simulink model "Experiment_4"  (R2018b)
settings: Solver=VariableStepAuto  StartTime=0.0  StopTime=2  RelTol=1e-3
libraries: dsparch4 x1, commsynccomp2 x1
settings Model: Creator=sangh  LastModifiedBy=sangh

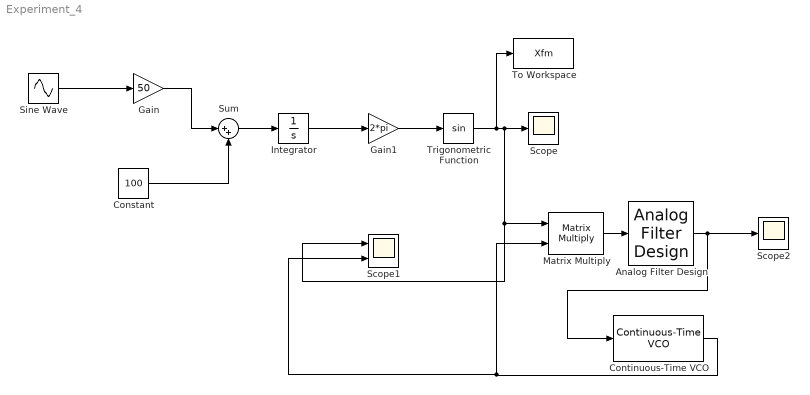
== system Experiment_4 ==
  Analog Filter Design : dsparch4/Analog Filter Design  method=Butterworth  filttype=Lowpass  N=5  Wlo=2*pi*10  Whi=80  Rp=2  Rs=40
  Constant : Constant  Value=100
  Continuous-Time VCO : commsynccomp2/Continuous-Time VCO  Ac=1  Fc=100  Kc=20  Ph=0
      settings: SourceProductName=Communications System Toolbox  SourceProductBaseCode=CM
  Gain : Gain  Gain=50
  Gain1 : Gain  Gain=2*pi
  Integrator : Integrator
  Matrix Multiply : Product  Multiplication=Matrix(*)
  Scope : Scope
  Scope1 : Scope  NumInputPorts=2
  Scope2 : Scope
  Sine Wave : Sin  Frequency=2*pi*10  SampleTime=1e-3
  Sum : Sum  Inputs=|++
  To Workspace : ToWorkspace  VariableName=Xfm  SampleTime=-1
  Trigonometric Function : Trigonometry
  wires:
  Sine Wave/1 -> Gain/1
  Gain/1 -> Sum/1
  Constant/1 -> Sum/2
  Sum/1 -> Integrator/1
  Integrator/1 -> Gain1/1
  Gain1/1 -> Trigonometric Function/1
  Trigonometric Function/1 -> To Workspace/1, Scope1/1, Matrix Multiply/1, Scope/1
  Matrix Multiply/1 -> Analog Filter Design/1
  Analog Filter Design/1 -> Continuous-Time VCO/1, Scope2/1
  Continuous-Time VCO/1 -> Scope1/2, Matrix Multiply/2
